simulink library "Lib_PFSys_ResistiveLine_TMATS"  (R2020b)
settings: Solver=ode45  StartTime=0.0  StopTime=10.0  RelTol=1e-3  EnableMultiTasking=on
libraries: Lib_PF_BusLoadDC_TMATS x1, Lib_PF_LineDC_TMATS x1
Description:
  | Thomas Modules
settings Model: Creator=jwchapm2  LastModifiedBy=bnakaya
settings DataIOCC: LimitDataPoints=on  SaveFormat=Array  ReturnWorkspaceOutputs=off
settings OptimizationCC: ExpressionDepthLimit=2147483647  LifeSpan=inf
settings DebuggingCC: UnderspecifiedInitializationDetection=Classic  MergeDetectMultiDrivingBlocksExec=none  SolverPrmCheckMsg=warning  StateNameClashWarn=warning  SFUnexpectedBacktrackingDiag=warning  SFNoUnconditionalDefaultTransitionDiag=warning  SFExecutionAtInitializationDiag=none  ArithmeticOperatorsInVariantConditions=warning
settings HardwareCC: ProdBitPerPointer=32  ProdBitPerSizeT=32  ProdBitPerPtrDiffT=32  ProdLargestAtomicFloat=None  ProdIntDivRoundTo=Undefined  ProdEndianess=Unspecified  ProdWordSize=32  ProdHWDeviceType=32-bit Generic
settings ModelReferenceCC: PropagateSignalLabelsOutOfModel=off
settings SFSimCC: SimUseLocalCustomCode=off  CustomCodeUndefinedFunction=UseInterfaceOnly
settings RTWCC: RTWUseLocalCustomCode=off
settings CodeAppCC: StateflowObjectComments=on
settings GRTTargetCC: TargetLangStandard=C89/C90 (ANSI)
settings ConfigComp: CovMetricSettings=dw  CovSaveCumulativeToWorkspaceVar=on  CovSaveSingleToWorkspaceVar=on  CovExternalEMLEnable=off

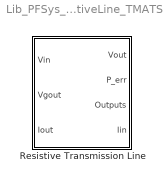
== system Lib_PFSys_ResistiveLine_TMATS ==
  Resistive Transmission Line : Subsystem  mask(Resistive Transmission Line){Z_M=0.001}
      mask prompts: Z_M "Z_M - Impedance"
      mask help: This block represents the resistive transmission line with a standar impedance of 0.001 Ohms.

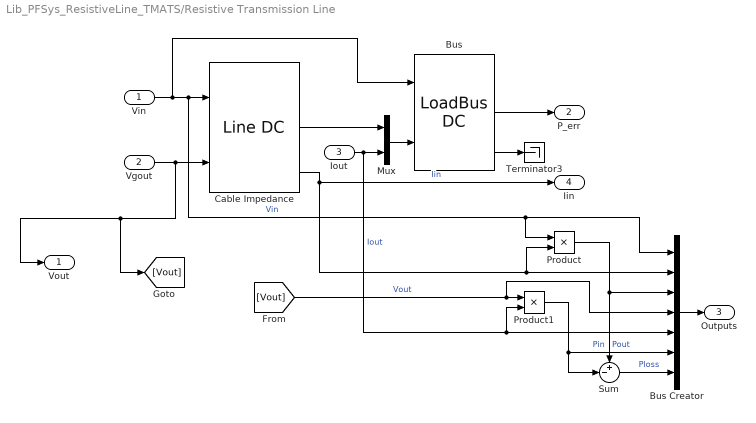
== system Lib_PFSys_ResistiveLine_TMATS/Resistive Transmission Line ==
  Vin : Inport
  Vgout : Inport  Port=2
  Iout : Inport  Port=3
  Bus : Lib_PF_BusLoadDC_TMATS/LoadBus DC  PeInEN_M=off  P_M=0  BlkNm_M=double(gcb)
  Bus Creator : BusCreator  Inputs=7
  Cable Impedance : Lib_PF_LineDC_TMATS/Line DC  R_M=Z_M
  Mux : Mux  Inputs=2
  Product : Product
  Product1 : Product
  Sum : Sum  Inputs=+-|
  Terminator3 : Terminator
  Vout : Outport
  P_err : Outport  Port=2
  Outputs : Outport  Port=3
  Iin : Outport  Port=4
  wires:
  Cable Impedance/2 -> Mux/1
  Sum/1 -> Bus Creator/7  "Ploss"
  Iout/1 -> Product1/2, Bus Creator/5, Mux/2  "Iout"
  [Vout] -> Bus Creator/4, Product1/1  "Vout"
  Product1/1 -> Bus Creator/6, Sum/2  "Pout"
  Cable Impedance/3 -> Product/2, Bus Creator/2, Iin/1  "Iin"
  Bus Creator/1 -> Outputs/1
  Vin/1 -> Bus/1, Cable Impedance/1, Product/1, Bus Creator/1  "Vin"
  Product/1 -> Bus Creator/3, Sum/1  "Pin"
  Mux/1 -> Bus/2
  Bus/3 -> Terminator3/1
  Vgout/1 -> [Vout], Vout/1, Cable Impedance/2
  Bus/2 -> P_err/1
